simulink model "PX4_Run_Mode_R2016b"  (R2017b)
settings: Solver=FixedStepDiscrete  StartTime=0.0  StopTime=inf  FixedStep=Ts  RelTol=1e-3  EnableMultiTasking=on
InitFcn:
  | run('InitFcn_R2016b.m');
values from neighbouring files (symbols this model uses):
  A = Pixhawk_CSC.Parameter( {single([diag([1 1 1]) Ts*diag([1 1 1]); diag([0 0 0]) diag([1 1 1])]),'A'} )    [InitFcn.m]    (also in InitFcn_R2016b.m; InitFcn_R2017b_no_csc.m = single([diag([1 1 1]) Ts*diag([1 1 1]); diag([0 0 0]) diag([)
  app = Pixhawk_CSC.Parameter({single( [0.05; 0.05; 0.05]),'app'} )    [InitFcn.m]    (also in InitFcn_R2016b.m; InitFcn_R2017b_no_csc.m = single( [0.05; 0.05; 0.05]))
  B = Pixhawk_CSC.Parameter( {single([Ts^2/2*diag([1 1 1]); Ts*diag([1 1 1])]),'B'} )    [InitFcn.m]    (also in InitFcn_R2016b.m; InitFcn_R2017b_no_csc.m = single([Ts^2/2*diag([1 1 1]); Ts*diag([1 1 1])]))
  Beta = Pixhawk_CSC.Parameter({single( 0.02),'Beta'} )    [InitFcn.m]    (also in InitFcn_R2016b.m; InitFcn_R2017b_no_csc.m = single( 0.02))
  C = Pixhawk_CSC.Parameter( {single([diag([1 1 1]) 0*diag([1 1 1]); zeros(1,2) 1 zeros(1,3)]),'C'} )    [InitFcn.m]    (also in InitFcn_R2016b.m; InitFcn_R2017b_no_csc.m = single([diag([1 1 1]) 0*diag([1 1 1]); zeros(1,2) 1 zeros(1,)
  C1 = Pixhawk_CSC.Parameter({single( 1.08680),'C1'} )    [InitFcn.m]    (also in InitFcn_R2016b.m; InitFcn_R2017b_no_csc.m = single( 1.08680))
  C10 = Pixhawk_CSC.Parameter({single( 0.0000),'C10'} )    [InitFcn.m]    (also in InitFcn_R2016b.m; InitFcn_R2017b_no_csc.m = single( 0.0000))
  C11 = Pixhawk_CSC.Parameter({single(-0.2300),'C11'} )    [InitFcn.m]    (also in InitFcn_R2016b.m; InitFcn_R2017b_no_csc.m = single(-0.2300))
  C12 = Pixhawk_CSC.Parameter({single( 0.0000),'C12'} )    [InitFcn.m]    (also in InitFcn_R2016b.m; InitFcn_R2017b_no_csc.m = single( 0.0000))
  C13 = Pixhawk_CSC.Parameter({single( 0.8000),'C13'} )    [InitFcn.m]    (also in InitFcn_R2016b.m; InitFcn_R2017b_no_csc.m = single( 0.8000))
  C14 = Pixhawk_CSC.Parameter({single( 0.8000),'C14'} )    [InitFcn.m]    (also in InitFcn_R2016b.m; InitFcn_R2017b_no_csc.m = single( 0.8000))
  C15 = Pixhawk_CSC.Parameter({single( 1.73200),'C15'} )    [InitFcn.m]    (also in InitFcn_R2016b.m; InitFcn_R2017b_no_csc.m = single( 1.73200))
  C16 = Pixhawk_CSC.Parameter({single( 0.1000),'C16'} )    [InitFcn.m]    (also in InitFcn_R2016b.m; InitFcn_R2017b_no_csc.m = single( 0.1000))
  C17 = Pixhawk_CSC.Parameter({single( 0.1000),'C17'} )    [InitFcn.m]    (also in InitFcn_R2016b.m; InitFcn_R2017b_no_csc.m = single( 0.1000))
  C18 = Pixhawk_CSC.Parameter({single( 0.0500),'C18'} )    [InitFcn.m]    (also in InitFcn_R2016b.m; InitFcn_R2017b_no_csc.m = single( 0.0500))
  C19 = Pixhawk_CSC.Parameter({single( 0.6000),'C19'} )    [InitFcn.m]    (also in InitFcn_R2016b.m; InitFcn_R2017b_no_csc.m = single( 0.6000))
  C2 = Pixhawk_CSC.Parameter({single( 1.10468),'C2'} )    [InitFcn.m]    (also in InitFcn_R2016b.m; InitFcn_R2017b_no_csc.m = single( 1.10468))
  C20 = Pixhawk_CSC.Parameter({single( 0.6000),'C20'} )    [InitFcn.m]    (also in InitFcn_R2016b.m; InitFcn_R2017b_no_csc.m = single( 0.6000))
  C21 = Pixhawk_CSC.Parameter({single( 1.04558),'C21'} )    [InitFcn.m]    (also in InitFcn_R2016b.m; InitFcn_R2017b_no_csc.m = single( 1.04558))
  C22 = Pixhawk_CSC.Parameter({single( 0.0000),'C22'} )    [InitFcn.m]    (also in InitFcn_R2016b.m; InitFcn_R2017b_no_csc.m = single( 0.0000))
  C23 = Pixhawk_CSC.Parameter({single( 0.0000),'C23'} )    [InitFcn.m]    (also in InitFcn_R2016b.m; InitFcn_R2017b_no_csc.m = single( 0.0000))
  C24 = Pixhawk_CSC.Parameter({single(-11.0000),'C24'} )    [InitFcn.m]    (also in InitFcn_R2016b.m; InitFcn_R2017b_no_csc.m = single(-11.0000))
  C3 = Pixhawk_CSC.Parameter({single( 1.1980),'C3'} )    [InitFcn.m]    (also in InitFcn_R2016b.m; InitFcn_R2017b_no_csc.m = single( 1.1980))
  C4 = Pixhawk_CSC.Parameter({single( 0.0500),'C4'} )    [InitFcn.m]    (also in InitFcn_R2016b.m; InitFcn_R2017b_no_csc.m = single( 0.0500))
  C5 = Pixhawk_CSC.Parameter({single( 0.0500),'C5'} )    [InitFcn.m]    (also in InitFcn_R2016b.m; InitFcn_R2017b_no_csc.m = single( 0.0500))
  C6 = Pixhawk_CSC.Parameter({single( 0.0500),'C6'} )    [InitFcn.m]    (also in InitFcn_R2016b.m; InitFcn_R2017b_no_csc.m = single( 0.0500))
  C7 = Pixhawk_CSC.Parameter({single( 0.35937),'C7'} )    [InitFcn.m]    (also in InitFcn_R2016b.m; InitFcn_R2017b_no_csc.m = single( 0.35937))
  C8 = Pixhawk_CSC.Parameter({single( 0.36528),'C8'} )    [InitFcn.m]    (also in InitFcn_R2016b.m; InitFcn_R2017b_no_csc.m = single( 0.36528))
  C9 = Pixhawk_CSC.Parameter({single( 0.53311),'C9'} )    [InitFcn.m]    (also in InitFcn_R2016b.m; InitFcn_R2017b_no_csc.m = single( 0.53311))
  C_1 = Pixhawk_CSC.Parameter( {single([diag([1 1 1]) 0*diag([1 1 1])]),'C1'} )    [InitFcn.m]    (also in InitFcn_R2016b.m; InitFcn_R2017b_no_csc.m = single([diag([1 1 1]) 0*diag([1 1 1])]))
  CAL_ACC0_XOFFSET = Pixhawk_CSC.Parameter( {single( 0.122052  ),'CAL_ACC0_XOFFSET'} )    [InitFcn.m]    (also in InitFcn_R2016b.m; InitFcn_R2017b_no_csc.m = single( 0.122052  ))
  CAL_ACC0_XXSCALE = Pixhawk_CSC.Parameter( {single(  1.01218    ),'CAL_ACC0_XXSCALE'} )    [InitFcn.m]    (also in InitFcn_R2016b.m; InitFcn_R2017b_no_csc.m = single(  1.01218    ))
  CAL_ACC0_XYSCALE = Pixhawk_CSC.Parameter( {single( -0.00443301 ),'CAL_ACC0_XYSCALE'} )    [InitFcn.m]    (also in InitFcn_R2016b.m; InitFcn_R2017b_no_csc.m = single( -0.00443301 ))
  CAL_ACC0_XZSCALE = Pixhawk_CSC.Parameter( {single( -0.00505793 ),'CAL_ACC0_XZSCALE'} )    [InitFcn.m]    (also in InitFcn_R2016b.m; InitFcn_R2017b_no_csc.m = single( -0.00505793 ))
  CAL_ACC0_YOFFSET = Pixhawk_CSC.Parameter( {single( 0.00281205),'CAL_ACC0_YOFFSET'} )    [InitFcn.m]    (also in InitFcn_R2016b.m; InitFcn_R2017b_no_csc.m = single( 0.00281205))
  CAL_ACC0_YXSCALE = Pixhawk_CSC.Parameter( {single( -0.00443301 ),'CAL_ACC0_YXSCALE'} )    [InitFcn.m]    (also in InitFcn_R2016b.m; InitFcn_R2017b_no_csc.m = single( -0.00443301 ))
  CAL_ACC0_YYSCALE = Pixhawk_CSC.Parameter( {single(  1.00234    ),'CAL_ACC0_YYSCALE'} )    [InitFcn.m]    (also in InitFcn_R2016b.m; InitFcn_R2017b_no_csc.m = single(  1.00234    ))
  CAL_ACC0_YZSCALE = Pixhawk_CSC.Parameter( {single(  0.0160883  ),'CAL_ACC0_YZSCALE'} )    [InitFcn.m]    (also in InitFcn_R2016b.m; InitFcn_R2017b_no_csc.m = single(  0.0160883  ))
  CAL_ACC0_ZOFFSET = Pixhawk_CSC.Parameter( {single(-0.0298121 ),'CAL_ACC0_ZOFFSET'} )    [InitFcn.m]    (also in InitFcn_R2016b.m; InitFcn_R2017b_no_csc.m = single(-0.0298121 ))
  CAL_ACC0_ZXSCALE = Pixhawk_CSC.Parameter( {single( -0.00505793 ),'CAL_ACC0_ZXSCALE'} )    [InitFcn.m]    (also in InitFcn_R2016b.m; InitFcn_R2017b_no_csc.m = single( -0.00505793 ))
  CAL_ACC0_ZYSCALE = Pixhawk_CSC.Parameter( {single(  0.0160883  ),'CAL_ACC0_ZYSCALE'} )    [InitFcn.m]    (also in InitFcn_R2016b.m; InitFcn_R2017b_no_csc.m = single(  0.0160883  ))
  CAL_ACC0_ZZSCALE = Pixhawk_CSC.Parameter( {single(  0.983604   ),'CAL_ACC0_ZZSCALE'} )    [InitFcn.m]    (also in InitFcn_R2016b.m; InitFcn_R2017b_no_csc.m = single(  0.983604   ))
  CAL_BAR_OFFSET = Pixhawk_CSC.Parameter( {single( -20.8468),'CAL_BAR_OFFSET'} )    [InitFcn.m]    (also in InitFcn_R2016b.m; InitFcn_R2017b_no_csc.m = single( -20.8468))
  CAL_BAR_SCALE = Pixhawk_CSC.Parameter( {single(   1.0632),'CAL_BAR_SCALE'} )    [InitFcn.m]    (also in InitFcn_R2016b.m; InitFcn_R2017b_no_csc.m = single(   1.0632))
  CAL_BAT0_XOFFSET = Pixhawk_CSC.Parameter( {single( 0.0000),'CAL_BAT0_XOFFSET'} )    [InitFcn.m]    (also in InitFcn_R2016b.m; InitFcn_R2017b_no_csc.m = single( 0.0000))
  CAL_BAT0_XXSCALE = Pixhawk_CSC.Parameter( {single(  1.0000),'CAL_BAT0_XXSCALE'} )    [InitFcn.m]    (also in InitFcn_R2016b.m; InitFcn_R2017b_no_csc.m = single(  1.0000))
  CAL_BAT0_XYSCALE = Pixhawk_CSC.Parameter( {single(  0.0000),'CAL_BAT0_XYSCALE'} )    [InitFcn.m]    (also in InitFcn_R2016b.m; InitFcn_R2017b_no_csc.m = single(  0.0000))
  CAL_BAT0_XZSCALE = Pixhawk_CSC.Parameter( {single(  0.0000),'CAL_BAT0_XZSCALE'} )    [InitFcn.m]    (also in InitFcn_R2016b.m; InitFcn_R2017b_no_csc.m = single(  0.0000))
  CAL_BAT0_YOFFSET = Pixhawk_CSC.Parameter( {single( 0.0000),'CAL_BAT0_YOFFSET'} )    [InitFcn.m]    (also in InitFcn_R2016b.m; InitFcn_R2017b_no_csc.m = single( 0.0000))
  CAL_BAT0_YXSCALE = Pixhawk_CSC.Parameter( {single(  0.0000),'CAL_BAT0_YXSCALE'} )    [InitFcn.m]    (also in InitFcn_R2016b.m; InitFcn_R2017b_no_csc.m = single(  0.0000))
  CAL_BAT0_YYSCALE = Pixhawk_CSC.Parameter( {single(  1.0000),'CAL_BAT0_YYSCALE'} )    [InitFcn.m]    (also in InitFcn_R2016b.m; InitFcn_R2017b_no_csc.m = single(  1.0000))
  CAL_BAT0_YZSCALE = Pixhawk_CSC.Parameter( {single(  0.0000),'CAL_BAT0_YZSCALE'} )    [InitFcn.m]    (also in InitFcn_R2016b.m; InitFcn_R2017b_no_csc.m = single(  0.0000))
  CAL_BAT0_ZOFFSET = Pixhawk_CSC.Parameter( {single( 0.0000),'CAL_BAT0_ZOFFSET'} )    [InitFcn.m]    (also in InitFcn_R2016b.m; InitFcn_R2017b_no_csc.m = single( 0.0000))
  CAL_BAT0_ZXSCALE = Pixhawk_CSC.Parameter( {single(  0.0000),'CAL_BAT0_ZXSCALE'} )    [InitFcn.m]    (also in InitFcn_R2016b.m; InitFcn_R2017b_no_csc.m = single(  0.0000))
  CAL_BAT0_ZYSCALE = Pixhawk_CSC.Parameter( {single(  0.0000),'CAL_BAT0_ZYSCALE'} )    [InitFcn.m]    (also in InitFcn_R2016b.m; InitFcn_R2017b_no_csc.m = single(  0.0000))
  CAL_BAT0_ZZSCALE = Pixhawk_CSC.Parameter( {single(  1.0000),'CAL_BAT0_ZZSCALE'} )    [InitFcn.m]    (also in InitFcn_R2016b.m; InitFcn_R2017b_no_csc.m = single(  1.0000))
  CAL_GPS0_XOFFSET = Pixhawk_CSC.Parameter( {single( 0.0000),'CAL_GPS0_XOFFSET'} )    [InitFcn.m]    (also in InitFcn_R2016b.m; InitFcn_R2017b_no_csc.m = single( 0.0000))
  CAL_GPS0_XXSCALE = Pixhawk_CSC.Parameter( {single(  0.0100),'CAL_GPS0_XXSCALE'} )    [InitFcn.m]    (also in InitFcn_R2016b.m; InitFcn_R2017b_no_csc.m = single(  0.0100))
  CAL_GPS0_XYSCALE = Pixhawk_CSC.Parameter( {single(  0.0000),'CAL_GPS0_XYSCALE'} )    [InitFcn.m]    (also in InitFcn_R2016b.m; InitFcn_R2017b_no_csc.m = single(  0.0000))
  CAL_GPS0_XZSCALE = Pixhawk_CSC.Parameter( {single(  0.0000),'CAL_GPS0_XZSCALE'} )    [InitFcn.m]    (also in InitFcn_R2016b.m; InitFcn_R2017b_no_csc.m = single(  0.0000))
  CAL_GPS0_YOFFSET = Pixhawk_CSC.Parameter( {single( 0.0000),'CAL_GPS0_YOFFSET'} )    [InitFcn.m]    (also in InitFcn_R2016b.m; InitFcn_R2017b_no_csc.m = single( 0.0000))
  CAL_GPS0_YXSCALE = Pixhawk_CSC.Parameter( {single(  0.0000),'CAL_GPS0_YXSCALE'} )    [InitFcn.m]    (also in InitFcn_R2016b.m; InitFcn_R2017b_no_csc.m = single(  0.0000))
  CAL_GPS0_YYSCALE = Pixhawk_CSC.Parameter( {single(  0.0100),'CAL_GPS0_YYSCALE'} )    [InitFcn.m]    (also in InitFcn_R2016b.m; InitFcn_R2017b_no_csc.m = single(  0.0100))
  CAL_GPS0_YZSCALE = Pixhawk_CSC.Parameter( {single(  0.0000),'CAL_GPS0_YZSCALE'} )    [InitFcn.m]    (also in InitFcn_R2016b.m; InitFcn_R2017b_no_csc.m = single(  0.0000))
  CAL_GPS0_ZOFFSET = Pixhawk_CSC.Parameter( {single( 0.0000),'CAL_GPS0_ZOFFSET'} )    [InitFcn.m]    (also in InitFcn_R2016b.m; InitFcn_R2017b_no_csc.m = single( 0.0000))
  CAL_GPS0_ZXSCALE = Pixhawk_CSC.Parameter( {single(  0.0000),'CAL_GPS0_ZXSCALE'} )    [InitFcn.m]    (also in InitFcn_R2016b.m; InitFcn_R2017b_no_csc.m = single(  0.0000))
  CAL_GPS0_ZYSCALE = Pixhawk_CSC.Parameter( {single(  0.0000),'CAL_GPS0_ZYSCALE'} )    [InitFcn.m]    (also in InitFcn_R2016b.m; InitFcn_R2017b_no_csc.m = single(  0.0000))
  CAL_GPS0_ZZSCALE = Pixhawk_CSC.Parameter( {single( -0.0010),'CAL_GPS0_ZZSCALE'} )    [InitFcn.m]    (also in InitFcn_R2016b.m; InitFcn_R2017b_no_csc.m = single( -0.0010))
  CAL_GYRO0_XXSCALE = Pixhawk_CSC.Parameter( {single(0.992736),'CAL_GYRO0_XXSCALE'} )    [InitFcn.m]    (also in InitFcn_R2016b.m; InitFcn_R2017b_no_csc.m = single(0.992736))
  CAL_GYRO0_XYSCALE = Pixhawk_CSC.Parameter( {single(0.0000),'CAL_GYRO0_XYSCALE'} )    [InitFcn.m]    (also in InitFcn_R2016b.m; InitFcn_R2017b_no_csc.m = single(0.0000))
  CAL_GYRO0_XZSCALE = Pixhawk_CSC.Parameter( {single(0.0000),'CAL_GYRO0_XZSCALE'} )    [InitFcn.m]    (also in InitFcn_R2016b.m; InitFcn_R2017b_no_csc.m = single(0.0000))
  CAL_GYRO0_YXSCALE = Pixhawk_CSC.Parameter( {single(0.0000),'CAL_GYRO0_YXSCALE'} )    [InitFcn.m]    (also in InitFcn_R2016b.m; InitFcn_R2017b_no_csc.m = single(0.0000))
  CAL_GYRO0_YYSCALE = Pixhawk_CSC.Parameter( {single(1.01609),'CAL_GYRO0_YYSCALE'} )    [InitFcn.m]    (also in InitFcn_R2016b.m; InitFcn_R2017b_no_csc.m = single(1.01609))
  CAL_GYRO0_YZSCALE = Pixhawk_CSC.Parameter( {single(0.0000),'CAL_GYRO0_YZSCALE'} )    [InitFcn.m]    (also in InitFcn_R2016b.m; InitFcn_R2017b_no_csc.m = single(0.0000))
  CAL_GYRO0_ZXSCALE = Pixhawk_CSC.Parameter( {single(0.0000),'CAL_GYRO0_ZXSCALE'} )    [InitFcn.m]    (also in InitFcn_R2016b.m; InitFcn_R2017b_no_csc.m = single(0.0000))
  CAL_GYRO0_ZYSCALE = Pixhawk_CSC.Parameter( {single(0.0000),'CAL_GYRO0_ZYSCALE'} )    [InitFcn.m]    (also in InitFcn_R2016b.m; InitFcn_R2017b_no_csc.m = single(0.0000))
  CAL_GYRO0_ZZSCALE = Pixhawk_CSC.Parameter( {single(1.03003),'CAL_GYRO0_ZZSCALE'} )    [InitFcn.m]    (also in InitFcn_R2016b.m; InitFcn_R2017b_no_csc.m = single(1.03003))
  CAL_MAG0_XCURCOR = Pixhawk_CSC.Parameter( {single( 0.0017     ),'CAL_MAG0_XCURCOR'} )    [InitFcn.m]    (also in InitFcn_R2016b.m; InitFcn_R2017b_no_csc.m = single( 0.0017     ))
  CAL_MAG0_XOFFSET = Pixhawk_CSC.Parameter( {single( 0.0446372  ),'CAL_MAG0_XOFFSET'} )    [InitFcn.m]    (also in InitFcn_R2016b.m; InitFcn_R2017b_no_csc.m = single( 0.0446372  ))
  CAL_MAG0_XXSCALE = Pixhawk_CSC.Parameter( {single(  1.01563   ),'CAL_MAG0_XXSCALE'} )    [InitFcn.m]    (also in InitFcn_R2016b.m; InitFcn_R2017b_no_csc.m = single(  1.01563   ))
  CAL_MAG0_XYSCALE = Pixhawk_CSC.Parameter( {single( -0.0612061 ),'CAL_MAG0_XYSCALE'} )    [InitFcn.m]    (also in InitFcn_R2016b.m; InitFcn_R2017b_no_csc.m = single( -0.0612061 ))
  CAL_MAG0_XZSCALE = Pixhawk_CSC.Parameter( {single( -0.011532  ),'CAL_MAG0_XZSCALE'} )    [InitFcn.m]    (also in InitFcn_R2016b.m; InitFcn_R2017b_no_csc.m = single( -0.011532  ))
  CAL_MAG0_YCURCOR = Pixhawk_CSC.Parameter( {single(-0.0075     ),'CAL_MAG0_YCURCOR'} )    [InitFcn.m]    (also in InitFcn_R2016b.m; InitFcn_R2017b_no_csc.m = single(-0.0075     ))
  CAL_MAG0_YOFFSET = Pixhawk_CSC.Parameter( {single( 0.0700776  ),'CAL_MAG0_YOFFSET'} )    [InitFcn.m]    (also in InitFcn_R2016b.m; InitFcn_R2017b_no_csc.m = single( 0.0700776  ))
  CAL_MAG0_YXSCALE = Pixhawk_CSC.Parameter( {single( -0.0612061 ),'CAL_MAG0_YXSCALE'} )    [InitFcn.m]    (also in InitFcn_R2016b.m; InitFcn_R2017b_no_csc.m = single( -0.0612061 ))
  CAL_MAG0_YYSCALE = Pixhawk_CSC.Parameter( {single(  1.00593   ),'CAL_MAG0_YYSCALE'} )    [InitFcn.m]    (also in InitFcn_R2016b.m; InitFcn_R2017b_no_csc.m = single(  1.00593   ))
  CAL_MAG0_YZSCALE = Pixhawk_CSC.Parameter( {single(  0.0144582 ),'CAL_MAG0_YZSCALE'} )    [InitFcn.m]    (also in InitFcn_R2016b.m; InitFcn_R2017b_no_csc.m = single(  0.0144582 ))
  CAL_MAG0_ZCURCOR = Pixhawk_CSC.Parameter( {single(-0.0080     ),'CAL_MAG0_ZCURCOR'} )    [InitFcn.m]    (also in InitFcn_R2016b.m; InitFcn_R2017b_no_csc.m = single(-0.0080     ))
  CAL_MAG0_ZOFFSET = Pixhawk_CSC.Parameter( {single( 0.00201742 ),'CAL_MAG0_ZOFFSET'} )    [InitFcn.m]    (also in InitFcn_R2016b.m; InitFcn_R2017b_no_csc.m = single( 0.00201742 ))
  CAL_MAG0_ZXSCALE = Pixhawk_CSC.Parameter( {single( -0.011532  ),'CAL_MAG0_ZXSCALE'} )    [InitFcn.m]    (also in InitFcn_R2016b.m; InitFcn_R2017b_no_csc.m = single( -0.011532  ))
  CAL_MAG0_ZYSCALE = Pixhawk_CSC.Parameter( {single(  0.0144582 ),'CAL_MAG0_ZYSCALE'} )    [InitFcn.m]    (also in InitFcn_R2016b.m; InitFcn_R2017b_no_csc.m = single(  0.0144582 ))
  CAL_MAG0_ZZSCALE = Pixhawk_CSC.Parameter( {single(  0.986813  ),'CAL_MAG0_ZZSCALE'} )    [InitFcn.m]    (also in InitFcn_R2016b.m; InitFcn_R2017b_no_csc.m = single(  0.986813  ))
  CAL_SONAR_OFFSET = Pixhawk_CSC.Parameter( {single( -6.8730),'CAL_SONAR_OFFSET'} )    [InitFcn.m]    (also in InitFcn_R2016b.m; InitFcn_R2017b_no_csc.m = single( -6.8730))
  CAL_SONAR_SCALE = Pixhawk_CSC.Parameter( {single(-438.1875),'CAL_SONAR_SCALE'} )    [InitFcn.m]    (also in InitFcn_R2016b.m; InitFcn_R2017b_no_csc.m = single(-438.1875))
  COM_RATE = double(10)    [InitFcn.m]    (also in InitFcn_R2016b.m; InitFcn_R2017b_no_csc.m)
  D = Pixhawk_CSC.Parameter( {single(zeros(size(C.Value,1), size(B.Value,2))),'D'} )    [InitFcn.m]    (also in InitFcn_R2016b.m; InitFcn_R2017b_no_csc.m = single(zeros(size(C,1), size(B,2))))
  Dip0 = Pixhawk_CSC.Parameter({single( 1.2),'Dip0'} )    [InitFcn.m]    (also in InitFcn_R2016b.m; InitFcn_R2017b_no_csc.m = single( 1.2))
  I = Pixhawk_CSC.Parameter( {single(eye(size(Q.Value))),'I'} )    [InitFcn.m]    (also in InitFcn_R2016b.m; InitFcn_R2017b_no_csc.m = single(eye(size(Q))))
  Jxx = Pixhawk_CSC.Parameter( {single(J(1,1)),'Jxx'} )    [InitFcn.m]    (also in InitFcn_R2016b.m; InitFcn_R2017b_no_csc.m = single(J(1,1)))
  Jyy = Pixhawk_CSC.Parameter( {single(J(2,2)),'Jyy'} )    [InitFcn.m]    (also in InitFcn_R2016b.m; InitFcn_R2017b_no_csc.m = single(J(2,2)))
  Jzz = Pixhawk_CSC.Parameter( {single(J(3,3)),'Jzz'} )    [InitFcn.m]    (also in InitFcn_R2016b.m; InitFcn_R2017b_no_csc.m = single(J(3,3)))
  Kapp = Pixhawk_CSC.Parameter({single( 1.2),'Kapp'} )    [InitFcn.m]    (also in InitFcn_R2016b.m; InitFcn_R2017b_no_csc.m = single( 1.2))
  Kx = Pixhawk_CSC.Parameter({single( Kx),'Kx'} )    [InitFcn.m]    (also in InitFcn_R2016b.m = Pixhawk_CSC.Parameter({single( [0.60 0.9]),'Kx'} ); InitFcn_R2017b_no_csc.m = single( [0.60 0.9]))
  Ky = Pixhawk_CSC.Parameter({single( Ky),'Ky'} )    [InitFcn.m]    (also in InitFcn_R2016b.m = Pixhawk_CSC.Parameter({single( [0.4 0.9]),'Ky'} ); InitFcn_R2017b_no_csc.m = single( [0.4 0.9]))
  LPF_REF_DEN = Pixhawk_CSC.Parameter( {single([1.0000 -0.8187]),'LPF_REF_DEN'} )    [InitFcn.m]    (also in InitFcn_R2016b.m; InitFcn_R2017b_no_csc.m = single([1.0000 -0.8187]))
  LPF_REF_NUM = Pixhawk_CSC.Parameter( {single([0.0000  0.1813]),'LPF_REF_NUM'} )    [InitFcn.m]    (also in InitFcn_R2016b.m; InitFcn_R2017b_no_csc.m = single([0.0000  0.1813]))
  m0 = Pixhawk_CSC.Parameter({single( 0.452857),'m0'} )    [InitFcn.m]    (also in InitFcn_R2016b.m; InitFcn_R2017b_no_csc.m = single( 0.452857))
  mn = [0.01; 0.01; 0.01; 0.01]    [InitFcn.m]    (also in InitFcn_R2016b.m; InitFcn_R2017b_no_csc.m)
  MOV_AVG_WINDOW = Pixhawk_CSC.Parameter( {single(100),'MOV_AVG_WINDOW'} )    [InitFcn.m]    (also in InitFcn_R2016b.m; InitFcn_R2017b_no_csc.m = single(100))
  Ox0 = Pixhawk_CSC.Parameter({single(O_x0),'Ox0'} )    [InitFcn.m]    (also in InitFcn_R2016b.m; InitFcn_R2017b_no_csc.m = single(O_x0))
  Oxa = Pixhawk_CSC.Parameter({single(O_x.a),'Oxa'} )    [InitFcn.m]    (also in InitFcn_R2016b.m; InitFcn_R2017b_no_csc.m = single(O_x.a))
  Oxb = Pixhawk_CSC.Parameter({single(O_x.b),'Oxb'} )    [InitFcn.m]    (also in InitFcn_R2016b.m; InitFcn_R2017b_no_csc.m = single(O_x.b))
  Oxc = Pixhawk_CSC.Parameter({single(O_x.c),'Oxc'} )    [InitFcn.m]    (also in InitFcn_R2016b.m; InitFcn_R2017b_no_csc.m = single(O_x.c))
  Oxd = Pixhawk_CSC.Parameter({single(O_x.d),'Oxd'} )    [InitFcn.m]    (also in InitFcn_R2016b.m; InitFcn_R2017b_no_csc.m = single(O_x.d))
  Oy0 = Pixhawk_CSC.Parameter({single(O_y0),'Oy0'} )    [InitFcn.m]    (also in InitFcn_R2016b.m; InitFcn_R2017b_no_csc.m = single(O_y0))
  Oya = Pixhawk_CSC.Parameter({single(O_y.a),'Oya'} )    [InitFcn.m]    (also in InitFcn_R2016b.m; InitFcn_R2017b_no_csc.m = single(O_y.a))
  Oyb = Pixhawk_CSC.Parameter({single(O_y.b),'Oyb'} )    [InitFcn.m]    (also in InitFcn_R2016b.m; InitFcn_R2017b_no_csc.m = single(O_y.b))
  Oyc = Pixhawk_CSC.Parameter({single(O_y.c),'Oyc'} )    [InitFcn.m]    (also in InitFcn_R2016b.m; InitFcn_R2017b_no_csc.m = single(O_y.c))
  Oyd = Pixhawk_CSC.Parameter({single(O_y.d),'Oyd'} )    [InitFcn.m]    (also in InitFcn_R2016b.m; InitFcn_R2017b_no_csc.m = single(O_y.d))
  Oz0 = Pixhawk_CSC.Parameter({single(O_z0),'Oz0'} )    [InitFcn.m]    (also in InitFcn_R2016b.m; InitFcn_R2017b_no_csc.m = single(O_z0))
  ... (+53 more)
undefined symbols (not defined in the file or in its folder): AccX, AccY, AccZ, Altitude, ax, ay, az, Current, FILTER_N, GPS_TS, GyroX, GyroY, GyroZ, Latitude, Longitude, M1_PWM, M2_PWM, M3_PWM, M4_PWM, MagX, MagY, MagZ, mAH, MOTOR, phi, Position_TS, psi, PX4_TUNE_ENUM, RGBLED_COLOR_ENUM, RGBLED_MODE_ENUM, S_AccX, S_AccY, S_AccZ, S_Altitude, S_Baro, S_Current, S_GyroX, S_GyroY, S_GyroZ, S_Latitude, S_Longitude, S_MagX, S_MagY, S_MagZ, S_mAH, S_N_Sat, S_Voltage, T_PITCH, T_ROLL, T_THROTTLE, theta, v, Voltage, w, wx, wxd, wy, wyd, wz ... (+4)
libraries: simulink x31, pixhawk_slib_sensors_actuators x7, pixhawk_slib_ADC_serial x5, pixhawk_slib_misc_utils x3, etargetslib x2
(part 2 of 7)

== system PX4_Run_Mode_R2016b/CONTROLLER/Inner Control Loop ==
  ESTIMATED_STATE_IN : Inport
  TARGET_IN : Inport  Port=2
  ERROR_IN : Inport  Port=3
  "SYSTEM_MODE_IN " : Inport  Port=4
  Pitch Control : Subsystem
  Roll Control : Subsystem
  Yaw Control : Subsystem
  ERROR_OUT : Outport
  U Roll : Outport  Port=2
  U Pitch : Outport  Port=3
  U Yaw : Outport  Port=4
  tag scope: TARGET=global
  wires:
  TARGET_IN/1 -> [TARGET], Roll Control/2(TARGET), Yaw Control/2(TARGET), Pitch Control/2(TARGET)
  ESTIMATED_STATE_IN/1 -> Yaw Control/3(ESTIMATED_STATE_IN), Roll Control/3(ESTIMATED_STATE_IN), Pitch Control/3(ESTIMATED_STATE_IN)
  Roll Control/1(U Roll) -> U Roll/1
  Pitch Control/1(U Pitch) -> U Pitch/1
  Yaw Control/1(U Yaw) -> U Yaw/1
  ERROR_IN/1 -> Roll Control/1(ERROR_IN)
  Roll Control/2(ERROR_OUT) -> Pitch Control/1(ERROR_IN)
  Pitch Control/2(ERROR_OUT) -> Yaw Control/1(ERROR_IN)
  Yaw Control/2(ERROR_OUT) -> ERROR_OUT/1
  "SYSTEM_MODE_IN "/1 -> Roll Control/4("SYSTEM_MODE_IN "), Pitch Control/4("SYSTEM_MODE_IN "), Yaw Control/4("SYSTEM_MODE_IN ")

== system PX4_Run_Mode_R2016b/CONTROLLER/Outer Control Loop ==
  ESTIMATED_STATE_IN : Inport
  TARGET_IN : Inport  Port=2
  SYSTEM_MODE_IN : Inport  Port=3
  Bus Assignment : BusAssignment  AssignedSignals=T_PITCH,T_ROLL,T_THROTTLE
  Bus Selector1 : BusSelector  OutputSignals=psi
  Bus Selector2 : BusSelector  OutputSignals=T_PITCH,T_ROLL,T_THROTTLE
  Bus Selector3 : BusSelector  OutputSignals=MAN_FLIGHT,SEMI_AUTO_FLIGHT,AUTO_FLIGHT
  Error Bus : Subsystem
  Flight_Mode_Selector : MATLAB Function  TreatAsAtomicUnit=on
  IMP Bus : Subsystem
  Thrust Control : Subsystem
  X Control : Subsystem
  Y Control : Subsystem
  TARGET_OUT : Outport
  ERROR_OUT : Outport  Port=2
  tag scope: IMP=global
  wires:
  TARGET_IN/1 -> Bus Selector2/1, Bus Assignment/1, Thrust Control/2(TARGET), Y Control/2(TARGET), X Control/2(TARGET)
  Bus Assignment/1 -> TARGET_OUT/1
  SYSTEM_MODE_IN/1 -> Bus Selector3/1, Thrust Control/4(SYSTEM_MODE_IN), Y Control/4(SYSTEM_MODE_IN), X Control/4(SYSTEM_MODE_IN)
  Bus Selector3/1 -> Flight_Mode_Selector/7(MANUAL_FLIGHT)  "<MAN_FLIGHT>"
  Bus Selector3/2 -> Flight_Mode_Selector/8(SEMI_AUTO_FLIGHT)  "<SEMI_AUTO_FLIGHT>"
  Bus Selector3/3 -> Flight_Mode_Selector/9(AUTO_FLIGHT)  "<AUTO_FLIGHT>"
  Bus Selector2/1 -> Flight_Mode_Selector/1(T_PITCH_IN)  "<T_PITCH>"
  Bus Selector2/2 -> Flight_Mode_Selector/2(T_ROLL_IN)  "<T_ROLL>"
  Bus Selector2/3 -> Flight_Mode_Selector/3(T_THROTTLE_IN)  "<T_THROTTLE>"
  Flight_Mode_Selector/1(T_PITCH_OUT) -> Bus Assignment/2
  Flight_Mode_Selector/2(T_ROLL_OUT) -> Bus Assignment/3
  Flight_Mode_Selector/3(T_THROTTLE_OUT) -> Bus Assignment/4
  Error Bus/1(ERROR_OUT) -> X Control/1(ERROR_IN)
  ESTIMATED_STATE_IN/1 -> Bus Selector1/1, Thrust Control/3(ESTIMATED_STATE_IN), Y Control/3(ESTIMATED_STATE_IN), X Control/3(ESTIMATED_STATE_IN)
  X Control/2(ERROR_OUT) -> Y Control/1(ERROR_IN)
  Y Control/2(ERROR_OUT) -> Thrust Control/1(ERROR_IN)
  Thrust Control/2(ERROR_OUT) -> ERROR_OUT/1
  Thrust Control/1(U Z) -> Flight_Mode_Selector/6(U_Z)
  Y Control/1(U Y) -> Flight_Mode_Selector/5(U_Y)
  X Control/1(U X) -> Flight_Mode_Selector/4(U_X)
  Bus Selector1/1 -> Flight_Mode_Selector/10(psi)  "<psi>"
  IMP Bus/1(IMP_OUT) -> [IMP]

== system PX4_Run_Mode_R2016b/CONTROLLER/Ramp ==
  SYSTEM_MODE_IN : Inport
  Bus Selector9 : BusSelector  OutputSignals=ARM_CMD,PRE_ARM_CMD
  Data Type Conversion13 : DataTypeConversion  OutDataTypeStr=single
  Digital Clock1 : DigitalClock  SampleTime=Ts
  Logical Operator2 : Logic  Operator=NOT  IconShape=distinctive  AllPortsSameDT=off  OutDataTypeStr=boolean
  Logical Operator3 : Logic  IconShape=distinctive  AllPortsSameDT=off  OutDataTypeStr=boolean
  Ramp1 : MATLAB Function  TreatAsAtomicUnit=on
  RAMP : Outport
  wires:
  SYSTEM_MODE_IN/1 -> Bus Selector9/1
  Bus Selector9/1 -> Logical Operator2/1  "<ARM_CMD>"
  Logical Operator2/1 -> Logical Operator3/1
  Bus Selector9/2 -> Logical Operator3/2  "<PRE_ARM_CMD>"
  Logical Operator3/1 -> Ramp1/2(Reset)
  Digital Clock1/1 -> Data Type Conversion13/1
  Data Type Conversion13/1 -> Ramp1/1(Clock)
  Ramp1/1(RAMP_OUT) -> RAMP/1

== system PX4_Run_Mode_R2016b/Communication System/Incomming Communication ==
  Byte Unpack1 : etargetslib/Byte Unpack  dimensions={[13]}  datatypes={'single'}  byteAlign=1
  Demux : Demux  Outputs=[1 12]
  MATLAB Function : MATLAB Function  TreatAsAtomicUnit=on
  Rate Transition1 : RateTransition  OutPortSampleTime=1/double(COM_RATE)
  Serial3 : pixhawk_slib_ADC_serial/Serial  DeviceName=/dev/ttyS2  ReadOrWrite=Reading  BaudRateStr=115200  block=off  WriteStatus=off  Terminator=off  Header=off  NumBytesRead=13*4+9  TerminatorChar=\n  HeaderData=[ uint8( hex2dec( 'DE' ) ), uint8( hex2dec( 'AD' ) ), uint8( hex2dec( 'C0' ) ), uint8( hex2dec( 'DE' ) ) ]  SimulateUsing=Code generation
      settings: SourceProductName=Pixhawk Target Blocks
  Serial5 : pixhawk_slib_ADC_serial/Serial  Commented=on  DeviceName=/dev/ttyACM0  ReadOrWrite=Reading  BaudRateStr=57600  block=off  WriteStatus=off  Terminator=off  Header=off  NumBytesRead=14*4+9  TerminatorChar=\n  HeaderData=[ uint8( hex2dec( 'DE' ) ), uint8( hex2dec( 'AD' ) ), uint8( hex2dec( 'C0' ) ), uint8( hex2dec( 'DE' ) ) ]  SimulateUsing=Code generation
      settings: SourceProductName=Pixhawk Target Blocks
  COM_IN : Outport
  Control Value : Outport  Port=2
  wires:
  MATLAB Function/1(y) -> Byte Unpack1/1
  Byte Unpack1/1 -> Rate Transition1/1
  Serial3/1 -> MATLAB Function/1(u)
  Rate Transition1/1 -> Demux/1
  Demux/2 -> COM_IN/1
  Demux/1 -> Control Value/1

== system PX4_Run_Mode_R2016b/Communication System/Outgoining Communication ==
  COM_OUT : Inport
  Byte Pack : etargetslib/Byte Pack  datatypes={'single'}  byteAlign=1
  Serial2 : pixhawk_slib_ADC_serial/Serial  DeviceName=/dev/ttyS2  ReadOrWrite=Writing  BaudRateStr=115200  block=off  WriteStatus=on  Terminator=off  Header=off  NumBytesRead=4  TerminatorChar=\n  HeaderData=[ uint8( hex2dec( 'DE' ) ), uint8( hex2dec( 'AD' ) ), uint8( hex2dec( 'C0' ) ), uint8( hex2dec( 'DE' ) ) ]  SimulateUsing=Code generation
      settings: SourceProductName=Pixhawk Target Blocks
  Serial4 : pixhawk_slib_ADC_serial/Serial  Commented=on  DeviceName=/dev/ttyACM0  ReadOrWrite=Writing  BaudRateStr=57600  block=off  WriteStatus=on  Terminator=off  Header=off  NumBytesRead=4  TerminatorChar=\n  HeaderData=[ uint8( hex2dec( 'DE' ) ), uint8( hex2dec( 'AD' ) ), uint8( hex2dec( 'C0' ) ), uint8( hex2dec( 'DE' ) ) ]  SimulateUsing=Code generation
      settings: SourceProductName=Pixhawk Target Blocks
  TrainStart : MATLAB Function  TreatAsAtomicUnit=on
  wires:
  Byte Pack/1 -> TrainStart/1(u)
  TrainStart/1(y) -> Serial2/1, Serial4/1
  COM_OUT/1 -> Byte Pack/1

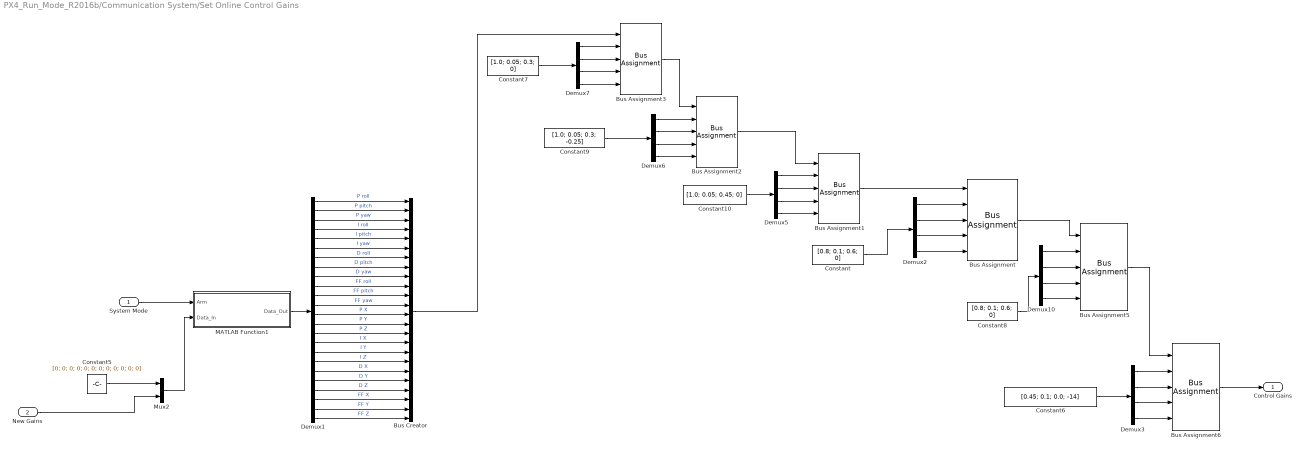
== system PX4_Run_Mode_R2016b/Communication System/Set Online Control Gains ==
  System Mode : Inport
  New Gains : Inport  Port=2
  Bus Assignment : BusAssignment  AssignedSignals=P X,I X,D X,FF X
  Bus Assignment1 : BusAssignment  AssignedSignals=P yaw,I yaw,D yaw,FF yaw
  Bus Assignment2 : BusAssignment  AssignedSignals=P pitch,I pitch,D pitch,FF pitch
  Bus Assignment3 : BusAssignment  AssignedSignals=P roll,I roll,D roll,FF roll
  Bus Assignment5 : BusAssignment  AssignedSignals=P Y,I Y,D Y,FF Y
  Bus Assignment6 : BusAssignment  AssignedSignals=P Z,I Z,D Z,FF Z
  Bus Creator : BusCreator  Inputs=24
  Constant : Constant  Value=[0.8; 0.1; 0.6; 0]  OutDataTypeStr=single  SampleTime=Ts
  Constant10 : Constant  Value=[1.0; 0.05; 0.45; 0]  OutDataTypeStr=single  SampleTime=Ts
  Constant5 : Constant  Value=[0; 0; 0; 0; 0; 0; 0; 0; 0; 0; 0; 0]  OutDataTypeStr=single
  Constant6 : Constant  Value=[0.45; 0.1; 0.0; -14]  OutDataTypeStr=single  SampleTime=Ts
  Constant7 : Constant  Value=[1.0; 0.05; 0.3; 0]  OutDataTypeStr=single  SampleTime=Ts
  Constant8 : Constant  Value=[0.8; 0.1; 0.6; 0]  OutDataTypeStr=single  SampleTime=Ts
  Constant9 : Constant  Value=[1.0; 0.05; 0.3; -0.25]  OutDataTypeStr=single  SampleTime=Ts
  Demux1 : Demux  Outputs=24
  Demux{2..3,5..7,10} (6 alike) : Demux
  MATLAB Function1 : MATLAB Function  TreatAsAtomicUnit=on
  Mux2 : Mux  Inputs=2
  Control Gains : Outport
  wires:
  Demux1/6 -> Bus Creator/6  "I yaw"
  Demux1/3 -> Bus Creator/3  "P yaw"
  Demux1/5 -> Bus Creator/5  "I pitch"
  Demux1/1 -> Bus Creator/1  "P roll"
  Demux1/2 -> Bus Creator/2  "P pitch"
  Demux1/4 -> Bus Creator/4  "I roll"
  Demux1/7 -> Bus Creator/7  "D roll"
  Demux1/8 -> Bus Creator/8  "D pitch"
  Demux1/9 -> Bus Creator/9  "D yaw"
  Demux1/11 -> Bus Creator/11  "FF pitch"
  Demux1/12 -> Bus Creator/12  "FF yaw"
  Demux1/10 -> Bus Creator/10  "FF roll"
  System Mode/1 -> MATLAB Function1/1(Arm)
  MATLAB Function1/1(Data_Out) -> Demux1/1
  Demux1/23 -> Bus Creator/23  "FF Y"
  Demux1/22 -> Bus Creator/22  "FF X"
  Demux1/21 -> Bus Creator/21  "D Z"
  Demux1/20 -> Bus Creator/20  "D Y"
  Demux1/19 -> Bus Creator/19  "D X"
  Demux1/18 -> Bus Creator/18  "I Z"
  Demux1/17 -> Bus Creator/17  "I Y"
  Demux1/16 -> Bus Creator/16  "I X"
  Demux1/15 -> Bus Creator/15  "P Z"
  Demux1/14 -> Bus Creator/14  "P Y"
  Demux1/13 -> Bus Creator/13  "P X"
  Demux1/24 -> Bus Creator/24  "FF Z"
  Constant/1 -> Demux2/1
  Demux2/2 -> Bus Assignment/3
  Demux2/1 -> Bus Assignment/2
  Demux2/3 -> Bus Assignment/4
  Bus Assignment1/1 -> Bus Assignment/1
  Demux5/1 -> Bus Assignment1/2
  Demux5/2 -> Bus Assignment1/3
  Demux5/3 -> Bus Assignment1/4
  Demux6/1 -> Bus Assignment2/2
  Demux6/2 -> Bus Assignment2/3
  Demux6/3 -> Bus Assignment2/4
  Constant9/1 -> Demux6/1
  Bus Assignment2/1 -> Bus Assignment1/1
  Demux7/1 -> Bus Assignment3/2
  Demux7/2 -> Bus Assignment3/3
  Demux7/3 -> Bus Assignment3/4
  Constant7/1 -> Demux7/1
  Bus Assignment3/1 -> Bus Assignment2/1
  Bus Creator/1 -> Bus Assignment3/1
  Bus Assignment/1 -> Bus Assignment5/1
  Demux10/1 -> Bus Assignment5/2
  Demux10/2 -> Bus Assignment5/3
  Demux10/3 -> Bus Assignment5/4
  Demux10/4 -> Bus Assignment5/5
  Constant8/1 -> Demux10/1
  Demux2/4 -> Bus Assignment/5
  Mux2/1 -> MATLAB Function1/2(Data_In)
  Bus Assignment5/1 -> Bus Assignment6/1
  Bus Assignment6/1 -> Control Gains/1
  Demux3/4 -> Bus Assignment6/5
  Demux3/3 -> Bus Assignment6/4
  Demux3/2 -> Bus Assignment6/3
  Demux3/1 -> Bus Assignment6/2
  Constant6/1 -> Demux3/1
  Constant5/1 -> Mux2/1
  New Gains/1 -> Mux2/2
  Demux5/4 -> Bus Assignment1/5
  Constant10/1 -> Demux5/1
  Demux6/4 -> Bus Assignment2/5
  Demux7/4 -> Bus Assignment3/5

== system PX4_Run_Mode_R2016b/Gathering Status for Logging Communication/ConvertM2Single ==
  M_IN : Inport
  Bus Creator1 : BusCreator  Inputs=7
  Bus to Vector1 : BusToVector
  Data Type Conversion1 : DataTypeConversion
  Demux : Demux  Outputs=7
  M_OUT : Outport
  wires:
  Bus to Vector1/1 -> Data Type Conversion1/1
  M_IN/1 -> Bus to Vector1/1
  Bus Creator1/1 -> M_OUT/1  "M"
  Data Type Conversion1/1 -> Demux/1
  Demux/2 -> Bus Creator1/2  "M2_PWM"
  Demux/3 -> Bus Creator1/3  "M3_PWM"
  Demux/1 -> Bus Creator1/1  "M1_PWM"
  Demux/4 -> Bus Creator1/4  "M4_PWM"
  Demux/5 -> Bus Creator1/5  "SOLVER_TYPE1"
  Demux/6 -> Bus Creator1/6  "SOLVER_TYPE2"
  Demux/7 -> Bus Creator1/7  "MOTOR"

== system PX4_Run_Mode_R2016b/Gathering Status for Logging Communication/ConvertM2Single1 ==
  SYSTEM_MODE_IN : Inport
  Bus Creator1 : BusCreator  Inputs=11
  Bus to Vector1 : BusToVector
  Data Type Conversion1 : DataTypeConversion
  Demux : Demux  Outputs=11
  SYSTEM_MODE_OUT : Outport
  wires:
  Bus to Vector1/1 -> Data Type Conversion1/1
  Bus Creator1/1 -> SYSTEM_MODE_OUT/1  "SYSTEM_MODE"
  Data Type Conversion1/1 -> Demux/1
  Demux/2 -> Bus Creator1/2  "PRE_ARM_CMD"
  Demux/3 -> Bus Creator1/3  "CONFIG_CMD"
  Demux/1 -> Bus Creator1/1  "ARM_CMD"
  Demux/4 -> Bus Creator1/4  "MAN_FLIGHR"
  SYSTEM_MODE_IN/1 -> Bus to Vector1/1
  Demux/5 -> Bus Creator1/5  "SEMI_AUTO_FLIGHT"
  Demux/6 -> Bus Creator1/6  "AUTO_FLIGHT"
  Demux/7 -> Bus Creator1/7  "RECORDING"
  Demux/8 -> Bus Creator1/8  "CONFIG_M1"
  Demux/9 -> Bus Creator1/9  "CONFIG_M2"
  Demux/10 -> Bus Creator1/10  "CONFIG_M3"
  Demux/11 -> Bus Creator1/11  "CONFIG_M4"

== system PX4_Run_Mode_R2016b/Gathering Status for Logging Communication/ConvertRC2Single ==
  RC_IN : Inport
  Bus Creator1 : BusCreator  Inputs=10
  Bus Selector : BusSelector  OutputSignals=Rc_Roll,Rc_Pitch,Rc_Yaw,Rc_Thrust,Rc_Arm,Rc_Config_1,Rc_Config_2,RC_Optional,Rc_RSSI,Rc_Failsafe
  Data Type Conversion{,1..9} (10 alike) : DataTypeConversion  OutDataTypeStr=single
  RC_OUT : Outport
  wires:
  Bus Creator1/1 -> RC_OUT/1  "RC"
  RC_IN/1 -> Bus Selector/1
  Bus Selector/1 -> Data Type Conversion/1  "<Rc_Roll>"
  Bus Selector/2 -> Data Type Conversion1/1  "<Rc_Pitch>"
  Bus Selector/3 -> Data Type Conversion2/1  "<Rc_Yaw>"
  Bus Selector/4 -> Data Type Conversion3/1  "<Rc_Thrust>"
  Bus Selector/5 -> Data Type Conversion4/1  "<Rc_Arm>"
  Bus Selector/6 -> Data Type Conversion5/1  "<Rc_Config_1>"
  Bus Selector/7 -> Data Type Conversion6/1  "<Rc_Config_2>"
  Bus Selector/9 -> Data Type Conversion7/1  "<Rc_RSSI>"
  Bus Selector/10 -> Data Type Conversion8/1  "<Rc_Failsafe>"
  Data Type Conversion/1 -> Bus Creator1/1  "RC_Roll"
  Data Type Conversion1/1 -> Bus Creator1/2  "RC_Pitch"
  Data Type Conversion2/1 -> Bus Creator1/3  "RC_Yaw"
  Data Type Conversion3/1 -> Bus Creator1/4  "RC_Thrust"
  Data Type Conversion4/1 -> Bus Creator1/5  "RC_Arm"
  Data Type Conversion5/1 -> Bus Creator1/6  "RC_Config_1"
  Data Type Conversion6/1 -> Bus Creator1/7  "RC_Config_2"
  Data Type Conversion7/1 -> Bus Creator1/9  "RC_RSSI"
  Data Type Conversion8/1 -> Bus Creator1/10  "RC_Failsafe"
  Bus Selector/8 -> Data Type Conversion9/1  "<RC_Optional>"
  Data Type Conversion9/1 -> Bus Creator1/8  "RC_Optional"

== system PX4_Run_Mode_R2016b/RC/Arming ==
  RC_INPUT : Inport
  Arming Conditions : simulink/Logic and Bit Operations/Compare To Constant  relop=>=  const=uint16(1333)  OutDataTypeStr=boolean
  Arming Conditions1 : simulink/Logic and Bit Operations/Compare To Constant  relop=<=  const=uint16(1666)  OutDataTypeStr=boolean
  Bus Selector : BusSelector  OutputSignals=Rc_Arm
  Config Conditions : simulink/Logic and Bit Operations/Compare To Constant  relop=>=  const=uint16(1666)  OutDataTypeStr=boolean
  Delay : Delay  DelayLength=MOV_AVG_WINDOW  InitialCondition=0  SampleTime=Ts
  Logical Operator1 : Logic  IconShape=distinctive  AllPortsSameDT=off  OutDataTypeStr=boolean
  Logical Operator2 : Logic  IconShape=distinctive  AllPortsSameDT=off  OutDataTypeStr=boolean
  Logical Operator3 : Logic  Operator=NOT  IconShape=distinctive  AllPortsSameDT=off  OutDataTypeStr=boolean
  Logical Operator8 : Logic  IconShape=distinctive  AllPortsSameDT=off  OutDataTypeStr=boolean
  ARM_CMD : Outport
  PRE_ARM_CMD : Outport  Port=2
  CONFIG_CMD : Outport  Port=3
  wires:
  Logical Operator8/1 -> Logical Operator2/1, Logical Operator1/2, Delay/1
  Arming Conditions1/1 -> Logical Operator8/2
  Arming Conditions/1 -> Logical Operator8/1
  Config Conditions/1 -> CONFIG_CMD/1
  Bus Selector/1 -> Config Conditions/1, Arming Conditions1/1, Arming Conditions/1  "<Rc_Arm>"
  Delay/1 -> Logical Operator1/1, Logical Operator3/1
  Logical Operator1/1 -> ARM_CMD/1
  RC_INPUT/1 -> Bus Selector/1
  Logical Operator3/1 -> Logical Operator2/2
  Logical Operator2/1 -> PRE_ARM_CMD/1

== system PX4_Run_Mode_R2016b/RC/Auto//Man Flight ==
  RC_INPUT : Inport
  Bus Selector3 : BusSelector  OutputSignals=Rc_Arm,Rc_Config_2
  Compare To Constant1 : simulink/Logic and Bit Operations/Compare To Constant  relop=>=  const=1666  OutDataTypeStr=boolean
  Compare To Constant3 : simulink/Logic and Bit Operations/Compare To Constant  relop=<=  const=1666  OutDataTypeStr=boolean
  Compare To Constant4 : simulink/Logic and Bit Operations/Compare To Constant  relop=>=  const=1333  OutDataTypeStr=boolean
  Compare To Constant5 : simulink/Logic and Bit Operations/Compare To Constant  relop=<=  const=1333  OutDataTypeStr=boolean
  Compare To Constant6 : simulink/Logic and Bit Operations/Compare To Constant  relop=>=  const=1333  OutDataTypeStr=boolean
  Compare To Constant7 : simulink/Logic and Bit Operations/Compare To Constant  relop=<=  const=1666  OutDataTypeStr=boolean
  Logical Operator1 : Logic  Inputs=3  IconShape=distinctive  AllPortsSameDT=off  OutDataTypeStr=boolean
  Logical Operator10 : Logic  Inputs=4  IconShape=distinctive  AllPortsSameDT=off  OutDataTypeStr=boolean
  Logical Operator9 : Logic  Inputs=3  IconShape=distinctive  AllPortsSameDT=off  OutDataTypeStr=boolean
  MANUAL_FLIGHT : Outport
  SEMI_AUTO_FLIGHT : Outport  Port=2
  AUTO_FLIGHT : Outport  Port=3
  wires:
  Compare To Constant4/1 -> Logical Operator1/2, Logical Operator10/2, Logical Operator9/2
  Logical Operator10/1 -> SEMI_AUTO_FLIGHT/1
  Compare To Constant3/1 -> Logical Operator10/1, Logical Operator1/1, Logical Operator9/1
  Bus Selector3/1 -> Compare To Constant3/1, Compare To Constant4/1  "<Rc_Arm>"
  Compare To Constant5/1 -> Logical Operator9/3
  Bus Selector3/2 -> Compare To Constant1/1, Compare To Constant7/1, Compare To Constant6/1, Compare To Constant5/1  "<Rc_Config_2>"
  Compare To Constant6/1 -> Logical Operator10/3
  Compare To Constant7/1 -> Logical Operator10/4
  Logical Operator9/1 -> MANUAL_FLIGHT/1
  RC_INPUT/1 -> Bus Selector3/1
  Logical Operator1/1 -> AUTO_FLIGHT/1
  Compare To Constant1/1 -> Logical Operator1/3

== system PX4_Run_Mode_R2016b/RC/Motor Configuration ==
  RC_INPUT : Inport
  Bus Selector2 : BusSelector  OutputSignals=Rc_Arm,Rc_Config_1,Rc_Config_2
  Config Conditions1 : simulink/Logic and Bit Operations/Compare To Constant  relop=>=  const=uint16(1666)  OutDataTypeStr=boolean
  Config Conditions2 : simulink/Logic and Bit Operations/Compare To Constant  relop=<=  const=uint16(1666)  OutDataTypeStr=boolean
  Config Conditions3 : simulink/Logic and Bit Operations/Compare To Constant  relop=>=  const=uint16(1333)  OutDataTypeStr=boolean
  Config Conditions4 : simulink/Logic and Bit Operations/Compare To Constant  relop=<=  const=uint16(1333)  OutDataTypeStr=boolean
  Config Conditions5 : simulink/Logic and Bit Operations/Compare To Constant  relop=<=  const=uint16(1666)  OutDataTypeStr=boolean
  Config Conditions6 : simulink/Logic and Bit Operations/Compare To Constant  relop=>=  const=uint16(1333)  OutDataTypeStr=boolean
  Config Conditions7 : simulink/Logic and Bit Operations/Compare To Constant  relop=<=  const=uint16(1333)  OutDataTypeStr=boolean
  Logical Operator1 : Logic  IconShape=distinctive  AllPortsSameDT=off  OutDataTypeStr=boolean
  Logical Operator{2..3,5,7} (4 alike) : Logic  Inputs=3  IconShape=distinctive  AllPortsSameDT=off  OutDataTypeStr=boolean
  Logical Operator6 : Logic  IconShape=distinctive  AllPortsSameDT=off  OutDataTypeStr=boolean
  CONFIG_M1 : Outport
  CONFIG_M2 : Outport  Port=2
  CONFIG_M3 : Outport  Port=3
  CONFIG_M4 : Outport  Port=4
  wires:
  Logical Operator3/1 -> CONFIG_M2/1  "CONFIG_M2"
  Logical Operator7/1 -> CONFIG_M4/1  "CONFIG_M4"
  Logical Operator2/1 -> CONFIG_M1/1  "CONFIG_M1"
  Bus Selector2/2 -> Config Conditions2/1, Config Conditions3/1, Config Conditions4/1  "<Rc_Config_1>"
  Logical Operator5/1 -> CONFIG_M3/1  "CONFIG_M3"
  Bus Selector2/1 -> Config Conditions1/1  "<Rc_Arm>"
  Config Conditions1/1 -> Logical Operator5/1, Logical Operator7/1, Logical Operator3/1, Logical Operator2/1
  Logical Operator6/1 -> Logical Operator3/3, Logical Operator7/3
  Logical Operator1/1 -> Logical Operator7/2, Logical Operator5/2
  RC_INPUT/1 -> Bus Selector2/1
  Config Conditions4/1 -> Logical Operator3/2, Logical Operator2/2
  Config Conditions3/1 -> Logical Operator1/1
  Config Conditions2/1 -> Logical Operator1/2
  Bus Selector2/3 -> Config Conditions5/1, Config Conditions6/1, Config Conditions7/1  "<Rc_Config_2>"
  Config Conditions6/1 -> Logical Operator6/1
  Config Conditions5/1 -> Logical Operator6/2
  Config Conditions7/1 -> Logical Operator2/3, Logical Operator5/3

== system PX4_Run_Mode_R2016b/RC/Recording Data ==
  RC_INPUT : Inport
  Bus Selector1 : BusSelector  OutputSignals=Rc_Arm,Rc_Config_1
  Compare To Constant1 : simulink/Logic and Bit Operations/Compare To Constant  relop=<=  const=1666  OutDataTypeStr=boolean
  Compare To Constant2 : simulink/Logic and Bit Operations/Compare To Constant  relop=>=  const=1333  OutDataTypeStr=boolean
  Logical Operator : Logic  IconShape=distinctive  AllPortsSameDT=off  OutDataTypeStr=boolean
  RECORDING : Outport
  wires:
  Bus Selector1/1 -> Compare To Constant1/1  "<Rc_Arm>"
  Compare To Constant1/1 -> Logical Operator/1
  Bus Selector1/2 -> Compare To Constant2/1  "<Rc_Config_1>"
  Compare To Constant2/1 -> Logical Operator/2
  RC_INPUT/1 -> Bus Selector1/1
  Logical Operator/1 -> RECORDING/1

== system PX4_Run_Mode_R2016b/SENSORS/Battery ==
  RAW_SENSOR_DATA_IN : Inport
  TIME_IN : Inport  Port=2
  Bus Assignment : BusAssignment  AssignedSignals=S_Voltage,S_Current,S_mAH
  Bus Assignment1 : BusAssignment  AssignedSignals=Battery_TS
  Data Type Conversion2 : DataTypeConversion  OutDataTypeStr=single
  battery_measure : pixhawk_slib_sensors_actuators/battery_measure  SampleTime=Ts  VoltageOut=on  VoltageFilteredOut=off  CurrentOut=on  mAH_Out=on  TimeStamp=on
      settings: SourceProductName=Pixhawk Target Blocks
  RAW_SENSOR_DATA_OUT : Outport
  TIME_OUT : Outport  Port=2
  wires:
  RAW_SENSOR_DATA_IN/1 -> Bus Assignment/1
  TIME_IN/1 -> Bus Assignment1/1
  Bus Assignment/1 -> RAW_SENSOR_DATA_OUT/1
  Bus Assignment1/1 -> TIME_OUT/1
  battery_measure/2 -> Bus Assignment/2
  battery_measure/3 -> Bus Assignment/3
  battery_measure/4 -> Bus Assignment/4
  battery_measure/1 -> Data Type Conversion2/1
  Data Type Conversion2/1 -> Bus Assignment1/2

== system PX4_Run_Mode_R2016b/SENSORS/Create Busses ==
  Bus Creator1 : BusCreator  Inputs=5
  Bus Creator2 : BusCreator  Inputs=18
  Constant : Constant  Value=[0; 0; 0; 0; 0; 0; 0; 0; 0; 0; 0; 0; 0; 0; 0; 0; 0; 0]  OutDataTypeStr=single  SampleTime=Ts
  Constant1 : Constant  Value=[0; 0; 0; 0; 0]  OutDataTypeStr=single  SampleTime=Ts
  Demux : Demux  Outputs=18
  Demux1 : Demux  Outputs=5
  RAW_SENSOR_DATA_OUT : Outport
  TIME_OUT : Outport  Port=2
  wires:
  Constant/1 -> Demux/1
  Demux/17 -> Bus Creator2/17  "S_mAH"
  Demux/8 -> Bus Creator2/8  "S_GyroY"
  Bus Creator2/1 -> RAW_SENSOR_DATA_OUT/1
  Demux/12 -> Bus Creator2/12  "S_Longitude"
  Demux/1 -> Bus Creator2/1  "S_MagX"
  Demux/9 -> Bus Creator2/9  "S_GyroZ"
  Demux/2 -> Bus Creator2/2  "S_MagY"
  Demux/15 -> Bus Creator2/15  "S_Voltage"
  Demux/7 -> Bus Creator2/7  "S_GyroX"
  Demux/16 -> Bus Creator2/16  "S_Current"
  Demux/13 -> Bus Creator2/13  "S_Altitude"
  Demux/5 -> Bus Creator2/5  "S_AccY"
  Demux/4 -> Bus Creator2/4  "S_AccX"
  Demux/6 -> Bus Creator2/6  "S_AccZ"
  Demux/3 -> Bus Creator2/3  "S_MagZ"
  Demux/11 -> Bus Creator2/11  "S_Latitude"
  Demux/10 -> Bus Creator2/10  "S_Baro"
  Demux/14 -> Bus Creator2/14  "S_N_Sat"
  Demux1/1 -> Bus Creator1/1  "Sensors_TS"
  Demux1/2 -> Bus Creator1/2  "Position_TS"
  Demux1/3 -> Bus Creator1/3  "GPS_TS"
  Demux1/4 -> Bus Creator1/4  "Battery_TS"
  Demux1/5 -> Bus Creator1/5  "Counter"
  Constant1/1 -> Demux1/1
  Bus Creator1/1 -> TIME_OUT/1
  Demux/18 -> Bus Creator2/18  "S_Sonar"

== system PX4_Run_Mode_R2016b/SENSORS/GPS ==
  RAW_SENSOR_DATA_IN : Inport
  TIME_IN : Inport  Port=2
  Bus Assignment : BusAssignment  AssignedSignals=S_Latitude,S_Longitude,S_Altitude,S_N_Sat
  Bus Assignment1 : BusAssignment  AssignedSignals=Position_TS,GPS_TS
  Data Type Conversion{,1..5} (6 alike) : DataTypeConversion  OutDataTypeStr=single
  vehicle_gps : pixhawk_slib_sensors_actuators/vehicle_gps  sampletime=Ts  show_ts_pos=on  show_alt=on  show_ts_gps=on  show_vel=off  show_fixtype=off  show_numsat=on
      settings: SourceProductName=Pixhawk Target Blocks
  RAW_SENSOR_DATA_OUT : Outport
  TIME_OUT : Outport  Port=2
  wires:
  RAW_SENSOR_DATA_IN/1 -> Bus Assignment/1
  TIME_IN/1 -> Bus Assignment1/1
  Bus Assignment/1 -> RAW_SENSOR_DATA_OUT/1
  Bus Assignment1/1 -> TIME_OUT/1
  vehicle_gps/1 -> Data Type Conversion/1
  vehicle_gps/2 -> Data Type Conversion1/1
  vehicle_gps/6 -> Data Type Conversion3/1
  vehicle_gps/4 -> Data Type Conversion2/1
  Data Type Conversion/1 -> Bus Assignment/2
  Data Type Conversion1/1 -> Bus Assignment/3
  Data Type Conversion2/1 -> Bus Assignment/4
  Data Type Conversion3/1 -> Bus Assignment/5
  vehicle_gps/5 -> Data Type Conversion4/1
  vehicle_gps/3 -> Data Type Conversion5/1
  Data Type Conversion4/1 -> Bus Assignment1/3
  Data Type Conversion5/1 -> Bus Assignment1/2

== system PX4_Run_Mode_R2016b/SENSORS/Sensor_Combined ==
  RAW_SENSOR_DATA_IN : Inport
  TIME_IN : Inport  Port=2
  Bus Assignment : BusAssignment  AssignedSignals=S_MagX,S_MagY,S_MagZ,S_AccX,S_AccY,S_AccZ,S_GyroX,S_GyroY,S_GyroZ,S_Baro
  Bus Assignment1 : BusAssignment  AssignedSignals=Sensors_TS
  Data Type Conversion2 : DataTypeConversion  OutDataTypeStr=single
  Gain : Gain  Gain=-1
  Gain1 : Gain  Gain=-1
  Gain2 : Gain  Gain=-1
  sensor_combined : pixhawk_slib_sensors_actuators/sensor_combined  sampletime=Ts  show_mag=on  show_acc=on  show_gyro=on  show_baro=on  show_ts=on
      settings: SourceProductName=Pixhawk Target Blocks
  RAW_SENSOR_DATA_OUT : Outport
  TIME_OUT : Outport  Port=2
  wires:
  RAW_SENSOR_DATA_IN/1 -> Bus Assignment/1
  TIME_IN/1 -> Bus Assignment1/1
  sensor_combined/4 -> Gain/1
  sensor_combined/5 -> Gain1/1
  sensor_combined/6 -> Gain2/1
  Bus Assignment/1 -> RAW_SENSOR_DATA_OUT/1
  sensor_combined/1 -> Bus Assignment/2
  sensor_combined/2 -> Bus Assignment/3
  sensor_combined/3 -> Bus Assignment/4
  Gain/1 -> Bus Assignment/5
  Gain1/1 -> Bus Assignment/6
  Gain2/1 -> Bus Assignment/7
  sensor_combined/7 -> Bus Assignment/8
  sensor_combined/8 -> Bus Assignment/9
  sensor_combined/9 -> Bus Assignment/10
  Bus Assignment1/1 -> TIME_OUT/1
  sensor_combined/11 -> Data Type Conversion2/1
  Data Type Conversion2/1 -> Bus Assignment1/2
  sensor_combined/10 -> Bus Assignment/11

== system PX4_Run_Mode_R2016b/SENSORS/Sonar ==
  RAW_SENSOR_DATA_IN : Inport
  TIME_IN : Inport  Port=2
  Bus Assignment : BusAssignment  AssignedSignals=S_Sonar
  Bus Assignment1 : BusAssignment  AssignedSignals=Counter
  Data Type Conversion17 : DataTypeConversion  OutDataTypeStr=single
  Data Type Conversion2 : DataTypeConversion  OutDataTypeStr=single
  Digital Clock : DigitalClock  SampleTime=Ts
  Read ADC Channels : pixhawk_slib_ADC_serial/Read ADC Channels  ADC_Channel_3_3_1=off  ADC_Channel_3_3_2=on  ADC_Channel_6_6=off  SampleTime=Ts  SimulateUsing=Code generation
      settings: SourceProductName=Pixhawk Target Blocks
  RAW_SENSOR_DATA_OUT : Outport
  TIME_OUT : Outport  Port=2
  wires:
  RAW_SENSOR_DATA_IN/1 -> Bus Assignment/1
  Bus Assignment/1 -> RAW_SENSOR_DATA_OUT/1
  TIME_IN/1 -> Bus Assignment1/1
  Read ADC Channels/1 -> Data Type Conversion17/1
  Data Type Conversion17/1 -> Bus Assignment/2
  Digital Clock/1 -> Data Type Conversion2/1
  Bus Assignment1/1 -> TIME_OUT/1
  Data Type Conversion2/1 -> Bus Assignment1/2
